simulink model "p2sim"  (R2017b)
settings: Solver=VariableStepAuto  StartTime=0.0  StopTime=2  RelTol=1e-3
values from neighbouring files (symbols this model uses):
  T = 0.25    [params.m]
undefined symbols (not defined in the file or in its folder): A1, B1, C1, D1
settings Model: Creator=Tomek  LastModifiedBy=Tomek

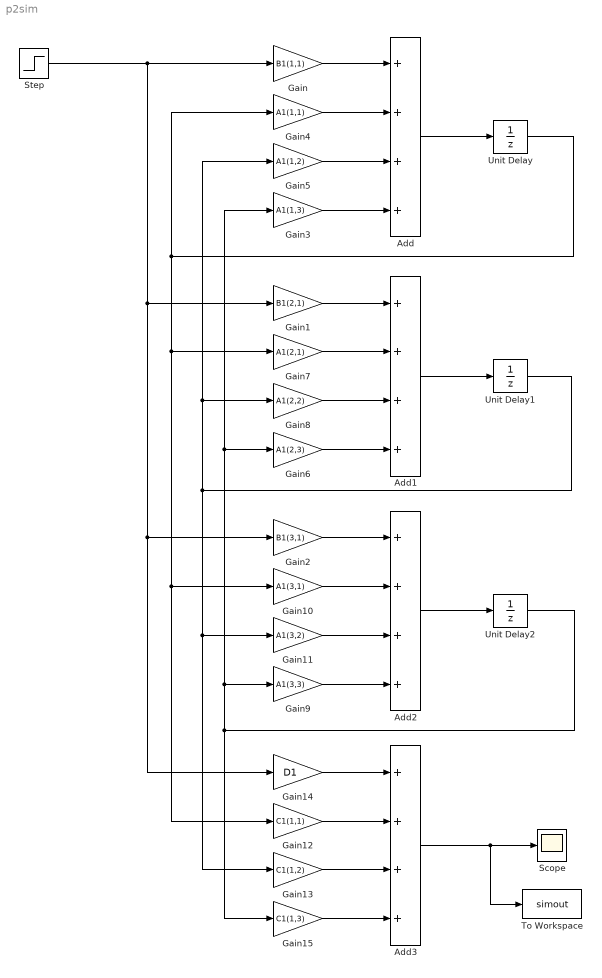
== system p2sim ==
  Add{,1..3} (4 alike) : Sum  Inputs=++++
  Gain : Gain  Gain=B1(1,1)
  Gain1 : Gain  Gain=B1(2,1)
  Gain10 : Gain  Gain=A1(3,1)
  Gain11 : Gain  Gain=A1(3,2)
  Gain12 : Gain  Gain=C1(1,1)
  Gain13 : Gain  Gain=C1(1,2)
  Gain14 : Gain  Gain=D1
  Gain15 : Gain  Gain=C1(1,3)
  Gain2 : Gain  Gain=B1(3,1)
  Gain3 : Gain  Gain=A1(1,3)
  Gain4 : Gain  Gain=A1(1,1)
  Gain5 : Gain  Gain=A1(1,2)
  Gain6 : Gain  Gain=A1(2,3)
  Gain7 : Gain  Gain=A1(2,1)
  Gain8 : Gain  Gain=A1(2,2)
  Gain9 : Gain  Gain=A1(3,3)
  Scope : Scope
  Step : Step  Before=-1  After=1100  SampleTime=0
  To Workspace : ToWorkspace  VariableName=simout  SaveFormat=Timeseries  SampleTime=-1
  Unit Delay : UnitDelay  SampleTime=T
  Unit Delay1 : UnitDelay  SampleTime=T
  Unit Delay2 : UnitDelay  SampleTime=T
  wires:
  Gain/1 -> Add/1
  Add/1 -> Unit Delay/1
  Gain4/1 -> Add/2
  Gain5/1 -> Add/3
  Gain3/1 -> Add/4
  Unit Delay/1 -> Gain10/1, Gain12/1, Gain7/1, Gain4/1
  Gain6/1 -> Add1/4
  Gain7/1 -> Add1/2
  Gain8/1 -> Add1/3
  Gain9/1 -> Add2/4
  Gain10/1 -> Add2/2
  Gain11/1 -> Add2/3
  Gain2/1 -> Add2/1
  Gain1/1 -> Add1/1
  Gain15/1 -> Add3/4
  Gain13/1 -> Add3/3
  Gain12/1 -> Add3/2
  Gain14/1 -> Add3/1
  Step/1 -> Gain14/1, Gain2/1, Gain1/1, Gain/1
  Add3/1 -> To Workspace/1, Scope/1
  Add1/1 -> Unit Delay1/1
  Add2/1 -> Unit Delay2/1
  Unit Delay2/1 -> Gain15/1, Gain3/1, Gain6/1, Gain9/1
  Unit Delay1/1 -> Gain13/1, Gain11/1, Gain5/1, Gain8/1
